simulink model "Model_mnogocanal_system_svyazi_s_code_razd_canalov"  (R2023b)
settings: Solver=VariableStepAuto  StartTime=0.0  StopTime=0.00001  RelTol=1e-3
libraries: simulink x12, dspfdesign x6
settings Model: Creator=User  LastModifiedBy=User

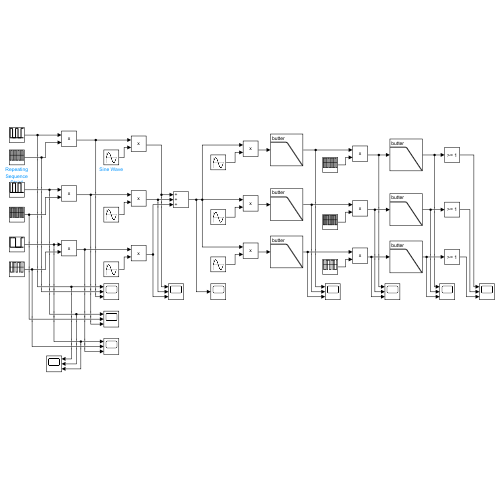
[thumbnail: Simulink's stored preview of the top-level diagram]
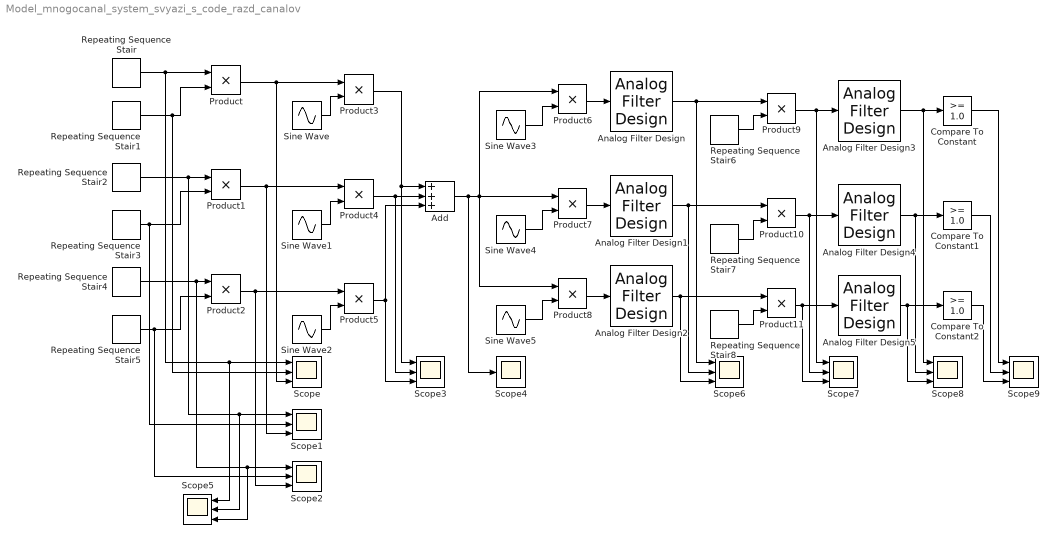
== system Model_mnogocanal_system_svyazi_s_code_razd_canalov ==
  Add : Sum  Inputs=+++
  Analog Filter Design{,1..5} (6 alike) : dspfdesign/Analog Filter Design  method=Butterworth  filttype=Lowpass  N=8  Wlo=30  Whi=80  Rp=2  Rs=40
  Compare To Constant : simulink/Logic and Bit Operations/Compare To Constant  relop=>=  const=1.0  OutDataTypeStr=boolean
  Compare To Constant1 : simulink/Logic and Bit Operations/Compare To Constant  relop=>=  const=1.0  OutDataTypeStr=boolean
  Compare To Constant2 : simulink/Logic and Bit Operations/Compare To Constant  relop=>=  const=1.0  OutDataTypeStr=boolean
  Product{,1..11} (12 alike) : Product
  Repeating Sequence Stair : simulink/Sources/Repeating Sequence Stair  OutValues=[1 0 1 0 1].'  tsamp=-1  OutMin=[]  OutMax=[]  OutDataTypeStr=double  OutputDataTypeScalingMode=double  OutDataType=fixdt(0,8)  ConRadixGroup=Best Precision: Vector-wise  OutScaling=2^-12
  Repeating Sequence Stair1 : simulink/Sources/Repeating Sequence Stair  OutValues=[1 -1 -1 1 1 -1 -1 1 1 -1 -1 1 1 -1 -1 1 1 -1 -1 1 1 -1 -1 1 1 -1 -1 1 1 -1 -1 1].'  tsamp=-1  OutMin=[]  OutMax=[]  OutDataTypeStr=double  OutputDataTypeScalingMode=double  OutDataType=fixdt(0,8)  ConRadixGroup=Best Precision: Vector-wise  OutScaling=2^-12
  Repeating Sequence Stair2 : simulink/Sources/Repeating Sequence Stair  OutValues=[0 1 0 1 0].'  tsamp=-1  OutMin=[]  OutMax=[]  OutDataTypeStr=double  OutputDataTypeScalingMode=double  OutDataType=fixdt(0,8)  ConRadixGroup=Best Precision: Vector-wise  OutScaling=2^-12
  Repeating Sequence Stair3 : simulink/Sources/Repeating Sequence Stair  OutValues=[1 -1 -1 1 -1 1 1 -1 -1 1 1 -1 1 -1 -1 1 1 -1 -1 1 -1 1 1 -1 -1 1 1 -1 1 -1 -1 1].'  tsamp=-1  OutMin=[]  OutMax=[]  OutDataTypeStr=double  OutputDataTypeScalingMode=double  OutDataType=fixdt(0,8)  ConRadixGroup=Best Precision: Vector-wise  OutScaling=2^-12
  Repeating Sequence Stair4 : simulink/Sources/Repeating Sequence Stair  OutValues=[1 1 0 0 1].'  tsamp=-1  OutMin=[]  OutMax=[]  OutDataTypeStr=double  OutputDataTypeScalingMode=double  OutDataType=fixdt(0,8)  ConRadixGroup=Best Precision: Vector-wise  OutScaling=2^-12
  Repeating Sequence Stair5 : simulink/Sources/Repeating Sequence Stair  OutValues=[1 1 -1 -1 -1 -1 1 1 -1 -1 1 1 1 1 -1 -1 -1 -1 1 1 1 1 -1 -1 1 1 -1 -1 -1 -1 1 1].'  tsamp=-1  OutMin=[]  OutMax=[]  OutDataTypeStr=double  OutputDataTypeScalingMode=double  OutDataType=fixdt(0,8)  ConRadixGroup=Best Precision: Vector-wise  OutScaling=2^-12
  Repeating Sequence Stair6 : simulink/Sources/Repeating Sequence Stair  OutValues=[1 -1 -1 1 1 -1 -1 1 1 -1 -1 1 1 -1 -1 1 1 -1 -1 1 1 -1 -1 1 1 -1 -1 1 1 -1 -1 1].'  tsamp=-1  OutMin=[]  OutMax=[]  OutDataTypeStr=double  OutputDataTypeScalingMode=double  OutDataType=fixdt(0,8)  ConRadixGroup=Best Precision: Vector-wise  OutScaling=2^-12
  Repeating Sequence Stair7 : simulink/Sources/Repeating Sequence Stair  OutValues=[1 -1 -1 1 -1 1 1 -1 -1 1 1 -1 1 -1 -1 1 1 -1 -1 1 -1 1 1 -1 -1 1 1 -1 1 -1 -1 1].'  tsamp=-1  OutMin=[]  OutMax=[]  OutDataTypeStr=double  OutputDataTypeScalingMode=double  OutDataType=fixdt(0,8)  ConRadixGroup=Best Precision: Vector-wise  OutScaling=2^-12
  Repeating Sequence Stair8 : simulink/Sources/Repeating Sequence Stair  OutValues=[1 1 -1 -1 -1 -1 1 1 -1 -1 1 1 1 1 -1 -1 -1 -1 1 1 1 1 -1 -1 1 1 -1 -1 -1 -1 1 1].'  tsamp=-1  OutMin=[]  OutMax=[]  OutDataTypeStr=double  OutputDataTypeScalingMode=double  OutDataType=fixdt(0,8)  ConRadixGroup=Best Precision: Vector-wise  OutScaling=2^-12
  Scope{,1..3,5..9} (9 alike) : Scope  NumInputPorts=3
  Scope4 : Scope
  Sine Wave : Sin  Frequency=500*10^3  SampleTime=0
  Sine Wave1 : Sin  Frequency=500*10^3  SampleTime=0
  Sine Wave2 : Sin  Frequency=500*10^3  SampleTime=0
  Sine Wave3 : Sin  Frequency=150*10^3  SampleTime=0
  Sine Wave4 : Sin  Frequency=150*10^3  SampleTime=0
  Sine Wave5 : Sin  Frequency=150*10^3  SampleTime=0
  wires:
  Repeating Sequence Stair/1 -> Product/1, Scope5/1, Scope/1
  Repeating Sequence Stair1/1 -> Product/2, Scope/2
  Repeating Sequence Stair2/1 -> Scope5/2, Scope1/1, Product1/1
  Repeating Sequence Stair3/1 -> Product1/2, Scope1/2
  Repeating Sequence Stair4/1 -> Scope5/3, Scope2/1, Product2/1
  Repeating Sequence Stair5/1 -> Product2/2, Scope2/2
  Product/1 -> Scope/3, Product3/1
  Product1/1 -> Scope1/3, Product4/1
  Product2/1 -> Scope2/3, Product5/1
  Sine Wave/1 -> Product3/2
  Sine Wave1/1 -> Product4/2
  Sine Wave2/1 -> Product5/2
  Sine Wave3/1 -> Product6/2
  Product4/1 -> Add/2, Scope3/2
  Product3/1 -> Add/1, Scope3/1
  Product5/1 -> Add/3, Scope3/3
  Sine Wave4/1 -> Product7/2
  Sine Wave5/1 -> Product8/2
  Product6/1 -> Analog Filter Design/1
  Product7/1 -> Analog Filter Design1/1
  Product8/1 -> Analog Filter Design2/1
  Analog Filter Design/1 -> Product9/1, Scope6/1
  Repeating Sequence Stair6/1 -> Product9/2
  Analog Filter Design1/1 -> Product10/1, Scope6/2
  Repeating Sequence Stair7/1 -> Product10/2
  Analog Filter Design2/1 -> Product11/1, Scope6/3
  Repeating Sequence Stair8/1 -> Product11/2
  Analog Filter Design3/1 -> Compare To Constant/1, Scope8/1
  Analog Filter Design4/1 -> Compare To Constant1/1, Scope8/2
  Analog Filter Design5/1 -> Compare To Constant2/1, Scope8/3
  Product9/1 -> Analog Filter Design3/1, Scope7/1
  Product10/1 -> Analog Filter Design4/1, Scope7/2
  Product11/1 -> Analog Filter Design5/1, Scope7/3
  Compare To Constant/1 -> Scope9/1
  Compare To Constant1/1 -> Scope9/2
  Compare To Constant2/1 -> Scope9/3
  Add/1 -> Scope4/1, Product6/1, Product8/1, Product7/1
